simulink model "MDCC"  (R2021b)
settings: Solver=FixedStepDiscrete  StartTime=0.0  StopTime=10.0  FixedStep=0.0001  RelTol=1e-3
model workspace (MATLAB code in the model file):
  | cmdLim = Simulink.Parameter;
  | cmdLim.Value = 15;
  | cmdLim.Description = 'Limit for controlling the maximum surface command angle.';
  | cmdLim.Min = 0;
  | cmdLim.Max = 90;
  | cmdLim.DocUnits = 'deg';
  | 
  | dispGain = Simulink.Parameter;
  | dispGain.Value = 0.75;
  | dispGain.Description = 'Gain applied to the displacement error.';
  | dispGain.Min = 0;
  | dispGain.Max = [];
  | dispGain.DocUnits = 'deg/sec/deg';
  | 
  | dispLim = Simulink.Parameter;
  | dispLim.Value = 30;
  | dispLim.Description = 'Limit for controlling the maximum commanded angle.';
  | dispLim.Min = 0;
  | dispLim.Max = 180;
  | dispLim.DocUnits = 'deg';
  | 
  | intGain = Simulink.Parameter;
  | intGain.Value = 0.5;
  | intGain.Description = 'Gain applied to the integral error.';
  | intGain.Min = 0;
  | intGain.Max = [];
  | intGain.DocUnits = 'deg/sec/deg/sec';
  | 
  | intLim = Simulink.Parameter;
  | intLim.Value = 5;
  | intLim.Description = 'Limit for controlling the maximum commanded angle.';
  | intLim.Min = 0;
  | intLim.Max = 90;
  | intLim.DocUnits = 'deg';
  | 
  | rateGain = Simulink.Parameter;
  | rateGain.Value = 2;
  | rateGain.Description = 'Gain applied to the rate error.';
  | rateGain.Min = 0;
  | rateGain.Max = [];
  | rateGain.DocUnits = 'deg/deg/sec';
  | 
  | rateLim = Simulink.Parameter;
  | rateLim.Value = 6;
  | rateLim.Description = 'Limit for controlling the maximum commanded angle.';
  | rateLim.Min = 0;
  | rateLim.Max = 180;
  | rateLim.DocUnits = 'deg/sec';
  | 
  | hdgGain = Simulink.Parameter;
  | hdgGain.Value = 0.015;
values from neighbouring files (symbols this model uses):
  KfDeadCompen_SetDeltaTime_us = myPackage.Parameter    [DeadCompen.m]
  Ts = 5E-6    (= 5e-06)    [iPMSM_data.m]
  VbDeadComp_SwtUseIsttrDes_flg = myPackage.Parameter    [DeadCompen.m]
  VfDeadCompen_ISttrDdeThdSwt_A = myPackage.Parameter    [DeadCompen.m]
  VfDeadCompen_ISttrIgbtThdSwt_A = myPackage.Parameter    [DeadCompen.m]
  VfDeadCompen_rDdeISttrHi_R = myPackage.Parameter    [DeadCompen.m]
  VfDeadCompen_rDdeISttrLo_R = myPackage.Parameter    [DeadCompen.m]
  VfDeadCompen_rIgbtISttrHi_R = myPackage.Parameter    [DeadCompen.m]
  VfDeadCompen_rIgbtISttrLo_R = myPackage.Parameter    [DeadCompen.m]
  VfDeadCompen_uDdeISttrHi_V = myPackage.Parameter    [DeadCompen.m]
  VfDeadCompen_uDdeISttrLo_V = myPackage.Parameter    [DeadCompen.m]
  VfDeadCompen_uIgbtISttrHi_V = myPackage.Parameter    [DeadCompen.m]
  VfDeadCompen_uIgbtISttrLo_V = myPackage.Parameter    [DeadCompen.m]
undefined symbols (not defined in the file or in its folder): CosTable12bit_Y, GLBCal_GLBCal_Kf_DCLinkOverVolErrThd_V, GLBCal_GLBCal_Kf_DCLinkUnderVolErrThd_V, GLBCal_GLBCal_Kf_EquiLd_NULL, GLBCal_GLBCal_Kf_EquiLq_NULL, GLBCal_GLBCal_Kf_MotorRatedSpeed_rpm, GLBCal_GLBCal_Kf_MotorSpeedHysteresis_Coef, GLBCal_Ke_MotorPolePairsNum_NULL, IoHwAbOpArg_PwmDutyCyclePhU_NULL, IoHwAbOpArg_PwmDutyCyclePhV_NULL, IoHwAbOpArg_PwmDutyCyclePhW_NULL, IoHwAbOpArg_PwmOutputEn, KbMDCC_DeadTimeCompEn_flg, KbMDCC_MCF_flgHarmInIsdqTab11ZR_flg, KbMDCC_MCF_flgHarmInIsdqTab13ZR_flg, KbMDCC_MCF_flgHarmInIsdqTab5ZR_flg, KbMDCC_MCF_flgHarmInIsdqTab7ZR_flg, KbMDCC_MCF_flgHarmInject_flg, KbMDCC_SetEAngleEn_flg, KbMDCC_UdUqFwOmit_flg, KfDeadCompen_CpPeriodTimesT_NULL, KfMDCC_ActiveDischargeIdCurVal_A, KfMDCC_ActiveDischargeIqCurVal_A, KfMDCC_DCLinkVolRate_coef, KfMDCC_DebugEAngleInit_rad, KfMDCC_DebugUalphaVolCmd_V, KfMDCC_DebugUbetaVolCmd_V, KfMDCC_DebugUdCmd_V, KfMDCC_DebugUqCmd_V, KfMDCC_DebugUsCmd_V, KfMDCC_DebugUsRate_V, KfMDCC_IMCResp_NULL, KfMDCC_IMCStab_NULL, KfMDCC_InvParkCpPeriodTimesT_NULL, KfMDCC_MCF_CircAge_NULL, KfMDCC_MCF_flgUse11Harm_flg, KfMDCC_MCF_flgUse13Harm_flg, KfMDCC_MCF_flgUse5Harm_flg, KfMDCC_MCF_flgUse7Harm_flg, KfMDCC_MCF_Harm1113FLParamSpeedThrd_rads, KfMDCC_MCF_Harm57FLParamSpeedThrd_rads, KfMDCC_MCF_HarmcofFltN_NULL, KfMDCC_MCF_HarmCpnAg_NULL, KfMDCC_MCF_HarmfLParaHigh_coef, KfMDCC_MCF_HarmfLParaLow_coef, KfMDCC_MCF_HarmIn1113ZRY_Trq_Nm, KfMDCC_MCF_HarmIn11_SpdLimHigh_rads, KfMDCC_MCF_HarmIn11_SpdLimLow_rads, KfMDCC_MCF_HarmIn11ZRY_Isd_A, KfMDCC_MCF_HarmIn11ZRY_Isq_A, KfMDCC_MCF_HarmIn13_SpdLimHigh_rads, KfMDCC_MCF_HarmIn13_SpdLimLow_rads, KfMDCC_MCF_HarmIn13ZRY_Isd_A, KfMDCC_MCF_HarmIn13ZRY_Isq_A, KfMDCC_MCF_HarmIn57ZRY_Trq_Nm, KfMDCC_MCF_HarmIn5_SpdLimHigh_rads, KfMDCC_MCF_HarmIn5_SpdLimLow_rads, KfMDCC_MCF_HarmIn5ZRY_Isd_A, KfMDCC_MCF_HarmIn5ZRY_Isq_A, KfMDCC_MCF_HarmIn7_SpdLimHigh_rads ... (+47)
libraries: simulink x40, PMSM_Library x3, mcbcontrolslib x1
(part 6 of 8)

== system MDCC/DoCurCtr_sys/MDCC/SVM_Calc/DeadComp_Sys/DeadCur_Calc/N_Select_Calc/Subsystem2/Subsystem ==
  VfPwmFreq_Hz : Inport
  Add5 : Sum  Commented=on
  Divide : Product  Inputs=*/
  KfDeadCompen_CpPeriodTimesT_NULL : Constant  Value=KfDeadCompen_CpPeriodTimesT_NULL  OutDataTypeStr=single
  KfMDCC_InvParkCpPeriodTimesT_NULL : Constant  Commented=on  Value=KfMDCC_InvParkCpPeriodTimesT_NULL
  TimeComp : Outport
  wires:
  VfPwmFreq_Hz/1 -> Divide/2
  Divide/1 -> TimeComp/1
  KfDeadCompen_CpPeriodTimesT_NULL/1 -> Divide/1

== system MDCC/DoCurCtr_sys/MDCC/SVM_Calc/DeadComp_Sys/DeadTime_Calc/Tavon_Calc/ia/If Action Subsystem ==
  Phase_Dyc : Inport
  uIgbt : Inport  Port=2
  uDde : Inport  Port=3
  uDcLink : Inport  Port=4
  Action Port : ActionPort  ActionPortLabel=if(u1 == 1)
  Add : Sum  Inputs=-+
  Add1 : Sum  Inputs=+-
  Add2 : Sum  Inputs=--+
  Constant : Constant  OutDataTypeStr=single
  Divide : Product  Inputs=*/
  Product : Product
  Product1 : Product
  "dycCorr " : Outport
  wires:
  Phase_Dyc/1 -> Product/1, Add/1
  uIgbt/1 -> Product/2, Add2/1
  uDde/1 -> Add2/2, Product1/2
  Add/1 -> Product1/1
  Constant/1 -> Add/2
  Product/1 -> Add1/1
  Product1/1 -> Add1/2
  uDcLink/1 -> Add2/3
  Add1/1 -> Divide/1
  Add2/1 -> Divide/2
  Divide/1 -> "dycCorr "/1

== system MDCC/DoCurCtr_sys/MDCC/SVM_Calc/DeadComp_Sys/DeadTime_Calc/Tavon_Calc/ia/If Action Subsystem1 ==
  Phase_Dyc : Inport
  uIgbt : Inport  Port=2
  uDde : Inport  Port=3
  uDcLink : Inport  Port=4
  Action Port : ActionPort  ActionPortLabel=else
  Add : Sum  Inputs=-+
  Add1 : Sum  Inputs=+-
  Add2 : Sum  Inputs=--+
  Constant : Constant  OutDataTypeStr=single
  Divide : Product  Inputs=*/
  Product : Product
  Product1 : Product
  "dycCorr " : Outport
  wires:
  Phase_Dyc/1 -> Product/1, Add/1
  uDde/1 -> Add2/1, Product/2
  uIgbt/1 -> Add2/2, Product1/2
  Add/1 -> Product1/1
  Constant/1 -> Add/2
  Product/1 -> Add1/1
  Product1/1 -> Add1/2
  uDcLink/1 -> Add2/3
  Add1/1 -> Divide/1
  Add2/1 -> Divide/2
  Divide/1 -> "dycCorr "/1

== system MDCC/DoCurCtr_sys/MDCC/SVM_Calc/DeadComp_Sys/DeadTime_Calc/Tavon_Calc/ia/uDdeCalc ==
  iPhaseAbs : Inport
  Compare To Constant : simulink/Logic and Bit Operations/Compare To Constant  relop=<  const=VfDeadCompen_ISttrDdeThdSwt_A  OutDataTypeStr=boolean
  If : If  IfExpression=u1 == 1
  If Action Subsystem : Subsystem  TreatAsAtomicUnit=on
  If Action Subsystem1 : Subsystem  TreatAsAtomicUnit=on
  Merge : Merge
  uDde : Outport
  wires:
  iPhaseAbs/1 -> [A], Compare To Constant/1
  If/2 -> If Action Subsystem1/Action
  Merge/1 -> uDde/1
  If/1 -> If Action Subsystem/Action
  If Action Subsystem/1(UDde) -> Merge/1
  Compare To Constant/1 -> If/1
  If Action Subsystem1/1(UDde) -> Merge/2
  [A] -> If Action Subsystem/1(iPhaseAbs)
  [A] -> If Action Subsystem1/1(iPhaseAbs)

== system MDCC/DoCurCtr_sys/MDCC/SVM_Calc/DeadComp_Sys/DeadTime_Calc/Tavon_Calc/ia/uIgbtCalc ==
  iPhaseAbs : Inport
  Compare To Constant : simulink/Logic and Bit Operations/Compare To Constant  relop=<  const=VfDeadCompen_ISttrIgbtThdSwt_A  OutDataTypeStr=boolean
  If : If  IfExpression=u1 == 0
  If Action Subsystem : Subsystem  TreatAsAtomicUnit=on
  If Action Subsystem1 : Subsystem  TreatAsAtomicUnit=on
  Merge : Merge
  uIgbt : Outport
  wires:
  iPhaseAbs/1 -> Compare To Constant/1, [B]
  If/2 -> If Action Subsystem1/Action
  Merge/1 -> uIgbt/1
  If/1 -> If Action Subsystem/Action
  If Action Subsystem/1(uIgbt) -> Merge/1
  Compare To Constant/1 -> If/1
  If Action Subsystem1/1(uIgbt) -> Merge/2
  [B] -> If Action Subsystem/1(iPhaseAbs)
  [B] -> If Action Subsystem1/1(iPhaseAbs)

== system MDCC/DoCurCtr_sys/MDCC/SVM_Calc/DeadComp_Sys/DeadTime_Calc/Tavon_Calc/ib/If Action Subsystem ==
  Phase_Dyc : Inport
  uIgbt : Inport  Port=2
  uDde : Inport  Port=3
  uDcLink : Inport  Port=4
  Action Port : ActionPort  ActionPortLabel=if(u1 == 1)
  Add : Sum  Inputs=-+
  Add1 : Sum  Inputs=+-
  Add2 : Sum  Inputs=--+
  Constant : Constant  OutDataTypeStr=single
  Divide : Product  Inputs=*/
  Product : Product
  Product1 : Product
  "dycCorr " : Outport
  wires:
  Phase_Dyc/1 -> Product/1, Add/1
  uIgbt/1 -> Product/2, Add2/1
  uDde/1 -> Add2/2, Product1/2
  Add/1 -> Product1/1
  Constant/1 -> Add/2
  Product/1 -> Add1/1
  Product1/1 -> Add1/2
  uDcLink/1 -> Add2/3
  Add1/1 -> Divide/1
  Add2/1 -> Divide/2
  Divide/1 -> "dycCorr "/1

== system MDCC/DoCurCtr_sys/MDCC/SVM_Calc/DeadComp_Sys/DeadTime_Calc/Tavon_Calc/ib/If Action Subsystem1 ==
  Phase_Dyc : Inport
  uIgbt : Inport  Port=2
  uDde : Inport  Port=3
  uDcLink : Inport  Port=4
  Action Port : ActionPort  ActionPortLabel=else
  Add : Sum  Inputs=-+
  Add1 : Sum  Inputs=+-
  Add2 : Sum  Inputs=--+
  Constant : Constant  OutDataTypeStr=single
  Divide : Product  Inputs=*/
  Product : Product
  Product1 : Product
  "dycCorr " : Outport
  wires:
  Phase_Dyc/1 -> Product/1, Add/1
  uDde/1 -> Add2/1, Product/2
  uIgbt/1 -> Add2/2, Product1/2
  Add/1 -> Product1/1
  Constant/1 -> Add/2
  Product/1 -> Add1/1
  Product1/1 -> Add1/2
  uDcLink/1 -> Add2/3
  Add1/1 -> Divide/1
  Add2/1 -> Divide/2
  Divide/1 -> "dycCorr "/1

== system MDCC/DoCurCtr_sys/MDCC/SVM_Calc/DeadComp_Sys/DeadTime_Calc/Tavon_Calc/ib/uDdeCalc ==
  iPhaseAbs : Inport
  Compare To Constant : simulink/Logic and Bit Operations/Compare To Constant  relop=<  const=VfDeadCompen_ISttrDdeThdSwt_A  OutDataTypeStr=boolean
  If : If  IfExpression=u1 == 1
  If Action Subsystem : Subsystem  TreatAsAtomicUnit=on
  If Action Subsystem1 : Subsystem  TreatAsAtomicUnit=on
  Merge : Merge
  uDde : Outport
  wires:
  iPhaseAbs/1 -> [A], Compare To Constant/1
  If/2 -> If Action Subsystem1/Action
  Merge/1 -> uDde/1
  If/1 -> If Action Subsystem/Action
  If Action Subsystem/1(UDde) -> Merge/1
  Compare To Constant/1 -> If/1
  If Action Subsystem1/1(UDde) -> Merge/2
  [A] -> If Action Subsystem/1(iPhaseAbs)
  [A] -> If Action Subsystem1/1(iPhaseAbs)

== system MDCC/DoCurCtr_sys/MDCC/SVM_Calc/DeadComp_Sys/DeadTime_Calc/Tavon_Calc/ib/uIgbtCalc ==
  iPhaseAbs : Inport
  Compare To Constant : simulink/Logic and Bit Operations/Compare To Constant  relop=<  const=VfDeadCompen_ISttrIgbtThdSwt_A  OutDataTypeStr=boolean
  If : If  IfExpression=u1 == 0
  If Action Subsystem : Subsystem  TreatAsAtomicUnit=on
  If Action Subsystem1 : Subsystem  TreatAsAtomicUnit=on
  Merge : Merge
  uIgbt : Outport
  wires:
  iPhaseAbs/1 -> Compare To Constant/1, [B]
  If/2 -> If Action Subsystem1/Action
  Merge/1 -> uIgbt/1
  If/1 -> If Action Subsystem/Action
  If Action Subsystem/1(uIgbt) -> Merge/1
  Compare To Constant/1 -> If/1
  If Action Subsystem1/1(uIgbt) -> Merge/2
  [B] -> If Action Subsystem/1(iPhaseAbs)
  [B] -> If Action Subsystem1/1(iPhaseAbs)

== system MDCC/DoCurCtr_sys/MDCC/SVM_Calc/DeadComp_Sys/DeadTime_Calc/Tavon_Calc/ic/If Action Subsystem ==
  Phase_Dyc : Inport
  uIgbt : Inport  Port=2
  uDde : Inport  Port=3
  uDcLink : Inport  Port=4
  Action Port : ActionPort  ActionPortLabel=if(u1 == 1)
  Add : Sum  Inputs=-+
  Add1 : Sum  Inputs=+-
  Add2 : Sum  Inputs=--+
  Constant : Constant  OutDataTypeStr=single
  Divide : Product  Inputs=*/
  Product : Product
  Product1 : Product
  "dycCorr " : Outport
  wires:
  Phase_Dyc/1 -> Product/1, Add/1
  uIgbt/1 -> Product/2, Add2/1
  uDde/1 -> Add2/2, Product1/2
  Add/1 -> Product1/1
  Constant/1 -> Add/2
  Product/1 -> Add1/1
  Product1/1 -> Add1/2
  uDcLink/1 -> Add2/3
  Add1/1 -> Divide/1
  Add2/1 -> Divide/2
  Divide/1 -> "dycCorr "/1

== system MDCC/DoCurCtr_sys/MDCC/SVM_Calc/DeadComp_Sys/DeadTime_Calc/Tavon_Calc/ic/If Action Subsystem1 ==
  Phase_Dyc : Inport
  uIgbt : Inport  Port=2
  uDde : Inport  Port=3
  uDcLink : Inport  Port=4
  Action Port : ActionPort  ActionPortLabel=else
  Add : Sum  Inputs=-+
  Add1 : Sum  Inputs=+-
  Add2 : Sum  Inputs=--+
  Constant : Constant  OutDataTypeStr=single
  Divide : Product  Inputs=*/
  Product : Product
  Product1 : Product
  "dycCorr " : Outport
  wires:
  Phase_Dyc/1 -> Product/1, Add/1
  uDde/1 -> Add2/1, Product/2
  uIgbt/1 -> Add2/2, Product1/2
  Add/1 -> Product1/1
  Constant/1 -> Add/2
  Product/1 -> Add1/1
  Product1/1 -> Add1/2
  uDcLink/1 -> Add2/3
  Add1/1 -> Divide/1
  Add2/1 -> Divide/2
  Divide/1 -> "dycCorr "/1

== system MDCC/DoCurCtr_sys/MDCC/SVM_Calc/DeadComp_Sys/DeadTime_Calc/Tavon_Calc/ic/uDdeCalc ==
  iPhaseAbs : Inport
  Compare To Constant : simulink/Logic and Bit Operations/Compare To Constant  relop=<  const=VfDeadCompen_ISttrDdeThdSwt_A  OutDataTypeStr=boolean
  If : If  IfExpression=u1 == 1
  If Action Subsystem : Subsystem  TreatAsAtomicUnit=on
  If Action Subsystem1 : Subsystem  TreatAsAtomicUnit=on
  Merge : Merge
  uDde : Outport
  wires:
  iPhaseAbs/1 -> [A], Compare To Constant/1
  If/2 -> If Action Subsystem1/Action
  Merge/1 -> uDde/1
  If/1 -> If Action Subsystem/Action
  If Action Subsystem/1(UDde) -> Merge/1
  Compare To Constant/1 -> If/1
  If Action Subsystem1/1(UDde) -> Merge/2
  [A] -> If Action Subsystem/1(iPhaseAbs)
  [A] -> If Action Subsystem1/1(iPhaseAbs)

== system MDCC/DoCurCtr_sys/MDCC/SVM_Calc/DeadComp_Sys/DeadTime_Calc/Tavon_Calc/ic/uIgbtCalc ==
  iPhaseAbs : Inport
  Compare To Constant : simulink/Logic and Bit Operations/Compare To Constant  relop=<  const=VfDeadCompen_ISttrIgbtThdSwt_A  OutDataTypeStr=boolean
  If : If  IfExpression=u1 == 0
  If Action Subsystem : Subsystem  TreatAsAtomicUnit=on
  If Action Subsystem1 : Subsystem  TreatAsAtomicUnit=on
  Merge : Merge
  uIgbt : Outport
  wires:
  iPhaseAbs/1 -> Compare To Constant/1, [B]
  If/2 -> If Action Subsystem1/Action
  Merge/1 -> uIgbt/1
  If/1 -> If Action Subsystem/Action
  If Action Subsystem/1(uIgbt) -> Merge/1
  Compare To Constant/1 -> If/1
  If Action Subsystem1/1(uIgbt) -> Merge/2
  [B] -> If Action Subsystem/1(iPhaseAbs)
  [B] -> If Action Subsystem1/1(iPhaseAbs)

== system MDCC/DoCurCtr_sys/MDCC/SVM_Calc/MDSA/SVM_PU/T1_T2_Calc/Subsystem1/Enabled Subsystem ==
  Z : Inport
  Y : Inport  Port=2
  Action Port : ActionPort  ActionPortLabel=case [ 1 ]:
  T4 : Outport
  T6 : Outport  Port=2
  wires:
  Z/1 -> T4/1
  Y/1 -> T6/1

== system MDCC/DoCurCtr_sys/MDCC/SVM_Calc/MDSA/SVM_PU/T1_T2_Calc/Subsystem1/Enabled Subsystem1 ==
  Y : Inport
  X : Inport  Port=2
  Action Port : ActionPort  ActionPortLabel=case [ 2 ]:
  Gain : Gain  Gain=-1
  T4 : Outport
  T6 : Outport  Port=2
  wires:
  Y/1 -> T4/1
  Gain/1 -> T6/1
  X/1 -> Gain/1

== system MDCC/DoCurCtr_sys/MDCC/SVM_Calc/MDSA/SVM_PU/T1_T2_Calc/Subsystem1/Enabled Subsystem2 ==
  Z : Inport
  X : Inport  Port=2
  Action Port : ActionPort  ActionPortLabel=case [ 3 ]:
  Gain : Gain  Gain=-1
  T4 : Outport
  T6 : Outport  Port=2
  wires:
  Z/1 -> Gain/1
  X/1 -> T6/1
  Gain/1 -> T4/1

== system MDCC/DoCurCtr_sys/MDCC/SVM_Calc/MDSA/SVM_PU/T1_T2_Calc/Subsystem1/Enabled Subsystem3 ==
  X : Inport
  Z : Inport  Port=2
  Action Port : ActionPort  ActionPortLabel=case [ 4 ]:
  Gain : Gain  Gain=-1
  T4 : Outport
  T6 : Outport  Port=2
  wires:
  X/1 -> Gain/1
  Z/1 -> T6/1
  Gain/1 -> T4/1

== system MDCC/DoCurCtr_sys/MDCC/SVM_Calc/MDSA/SVM_PU/T1_T2_Calc/Subsystem1/Enabled Subsystem4 ==
  X : Inport
  Y : Inport  Port=2
  Action Port : ActionPort  ActionPortLabel=case [ 5 ]:
  Gain : Gain  Gain=-1
  T4 : Outport
  T6 : Outport  Port=2
  wires:
  Y/1 -> Gain/1
  X/1 -> T4/1
  Gain/1 -> T6/1

== system MDCC/DoCurCtr_sys/MDCC/SVM_Calc/MDSA/SVM_PU/T1_T2_Calc/Subsystem1/Enabled Subsystem5 ==
  Y : Inport
  Z : Inport  Port=2
  Action Port : ActionPort  ActionPortLabel=case [ 6 ]:
  Gain : Gain  Gain=-1
  Gain1 : Gain  Gain=-1
  T4 : Outport
  T6 : Outport  Port=2
  wires:
  Y/1 -> Gain/1
  Z/1 -> Gain1/1
  Gain/1 -> T4/1
  Gain1/1 -> T6/1

== system MDCC/DoCurCtr_sys/MDCC/SVM_Calc/MDSA/SVM_PU/T1_T2_Calc/Subsystem1/Enabled Subsystem6 ==
  Y : Inport
  Z : Inport  Port=2
  Action Port : ActionPort  ActionPortLabel=default:
  Gain : Gain  Gain=-1
  Gain1 : Gain  Gain=-1
  T4 : Outport
  T6 : Outport  Port=2
  wires:
  Y/1 -> Gain/1
  Z/1 -> Gain1/1
  Gain/1 -> T4/1
  Gain1/1 -> T6/1

== system MDCC/DoCurCtr_sys/MDCC/SVM_Calc/MDSA/SVM_PU/T1_T2_Calc/Subsystem2/If Action Subsystem ==
  Bus_T4T6 : Inport
  Action Port : ActionPort  ActionPortLabel=else
  Bus Selector : BusSelector  OutputSignals=T4,T6
  Signal Copy1 : SignalConversion  OverrideOpt=off
  Signal Copy2 : SignalConversion  OverrideOpt=off
  T1 : Outport
  T2 : Outport  Port=2
  wires:
  Bus_T4T6/1 -> Bus Selector/1
  Bus Selector/1 -> Signal Copy1/1  "<T4>"
  Bus Selector/2 -> Signal Copy2/1  "<T6>"
  Signal Copy1/1 -> T1/1
  Signal Copy2/1 -> T2/1

== system MDCC/DoCurCtr_sys/MDCC/SVM_Calc/MDSA/SVM_PU/T1_T2_Calc/Subsystem2/If Action Subsystem1 ==
  Bus_T4T6 : Inport
  Action Port : ActionPort  ActionPortLabel=elseif(u1 > 1)
  Add : Sum
  Bus Selector : BusSelector  OutputSignals=T4,T6
  Divide : Product  Inputs=*/
  Divide1 : Product  Inputs=/*
  T1 : Outport
  T2 : Outport  Port=2
  wires:
  Bus_T4T6/1 -> Bus Selector/1
  Bus Selector/1 -> Divide/1, Add/1  "<T4>"
  Bus Selector/2 -> Divide1/2, Add/2  "<T6>"
  Add/1 -> Divide1/1, Divide/2
  Divide/1 -> T1/1  "T1"
  Divide1/1 -> T2/1  "T2"

== system MDCC/DoCurCtr_sys/MDCC/SVM_Calc/MDSA/SVM_PU/T1_T2_Calc/Subsystem2/If Action Subsystem2 ==
  Bus_T4T6 : Inport
  Action Port : ActionPort  ActionPortLabel=if(u1 > 1.154 )
  Add1 : Sum
  Add2 : Sum  Inputs=++-
  Bus Selector1 : BusSelector  OutputSignals=T4,T6
  Constant : Constant  Value=1.154  OutDataTypeStr=single
  Divide : Product  Inputs=*/
  Divide1 : Product  Inputs=/*
  If Action Subsystem2 : Subsystem  TreatAsAtomicUnit=on
  If Action Subsystem3 : Subsystem  TreatAsAtomicUnit=on
  If1 : If  IfExpression=u1 ~= 0
  Merge2 : Merge
  Merge3 : Merge
  Relational Operator1 : RelationalOperator  OutDataTypeStr=boolean  RndMeth=Simplest
  T1 : Outport
  T2 : Outport  Port=2
  wires:
  Bus_T4T6/1 -> Bus Selector1/1
  Bus Selector1/2 -> Divide1/2, Add2/2, Add1/2  "<T6>"
  Divide/1 -> [T4_m], Relational Operator1/1  "T4_m"
  Bus Selector1/1 -> Divide/1, Add2/1, Add1/1  "<T4>"
  Divide1/1 -> [T6_m], Relational Operator1/2  "T6_m"
  Add1/1 -> Divide1/1, Divide/2
  Relational Operator1/1 -> If1/1
  Constant/1 -> Add2/3
  Add2/1 -> If Action Subsystem2/3(delta), If Action Subsystem3/3(delta)  "delta"
  If1/1 -> If Action Subsystem2/Action
  If1/2 -> If Action Subsystem3/Action
  If Action Subsystem2/1(T1) -> Merge2/1
  If Action Subsystem3/1(T1) -> Merge2/2
  If Action Subsystem3/2(T2) -> Merge3/2
  If Action Subsystem2/2(T2) -> Merge3/1
  Merge2/1 -> T1/1  "T1"
  Merge3/1 -> T2/1  "T2"
  [T4_m] -> If Action Subsystem3/1(T4_m), If Action Subsystem2/1(T4_m)
  [T6_m] -> If Action Subsystem3/2(T6_m), If Action Subsystem2/2(T6_m)

== system MDCC/DoCurCtr_sys/MDCC/SVM_Calc/MDSA/SVPWM/vIntp_PWMFOC_CalSec/CalABC/CalA ==
  In1 : Inport
  Constant : Constant
  Constant1 : Constant  Value=0
  Data Type Conversion : DataTypeConversion
  Data Type Conversion1 : DataTypeConversion
  Switch : Switch  Criteria=u2 > Threshold  ZeroCross=off
  A : Outport
  wires:
  Switch/1 -> A/1
  Data Type Conversion1/1 -> Switch/3
  Data Type Conversion/1 -> Switch/1
  Constant1/1 -> Data Type Conversion1/1
  Constant/1 -> Data Type Conversion/1
  In1/1 -> Switch/2

== system MDCC/DoCurCtr_sys/MDCC/SVM_Calc/MDSA/SVPWM/vIntp_PWMFOC_CalSec/CalABC/CalB ==
  In1 : Inport
  Constant : Constant
  Constant1 : Constant  Value=0
  Data Type Conversion : DataTypeConversion
  Data Type Conversion1 : DataTypeConversion
  Switch : Switch  Criteria=u2 > Threshold  ZeroCross=off
  B : Outport
  wires:
  In1/1 -> Switch/2
  Constant/1 -> Data Type Conversion/1
  Constant1/1 -> Data Type Conversion1/1
  Data Type Conversion/1 -> Switch/1
  Data Type Conversion1/1 -> Switch/3
  Switch/1 -> B/1

== system MDCC/DoCurCtr_sys/MDCC/SVM_Calc/MDSA/SVPWM/vIntp_PWMFOC_CalSec/CalABC/CalC ==
  In1 : Inport
  Constant : Constant
  Constant1 : Constant  Value=0
  Data Type Conversion : DataTypeConversion
  Data Type Conversion1 : DataTypeConversion
  Switch : Switch  Criteria=u2 > Threshold  ZeroCross=off
  C : Outport
  wires:
  Switch/1 -> C/1
  Data Type Conversion1/1 -> Switch/3
  Data Type Conversion/1 -> Switch/1
  Constant1/1 -> Data Type Conversion1/1
  Constant/1 -> Data Type Conversion/1
  In1/1 -> Switch/2

== system MDCC/DoCurCtr_sys/MDCC/SVM_Calc/MDSA/SVPWM/vIntp_PWMFOC_CalSec/CalVaVbVc/CalVa ==
  In1 : Inport
  Bus Selector : BusSelector  OutputSignals=Ubeta
  Va : Outport
  wires:
  Bus Selector/1 -> Va/1  "<Ubeta>"
  In1/1 -> Bus Selector/1

== system MDCC/DoCurCtr_sys/MDCC/SVM_Calc/MDSA/SVPWM/vIntp_PWMFOC_CalSec/CalVaVbVc/CalVb ==
  In1 : Inport
  1/2 : Constant  Value=0.5
  Add : Sum  Inputs=+-
  Bus Selector : BusSelector  OutputSignals=Ualpha,Ubeta
  Data Type Conversion : DataTypeConversion
  Data Type Conversion1 : DataTypeConversion
  Data Type Conversion2 : DataTypeConversion
  Product1 : Product
  Product2 : Product
  Sqrt(3)/2 : Constant  Value=0.866025
  Vb : Outport
  wires:
  Data Type Conversion2/1 -> Vb/1
  Product1/1 -> Add/2
  Product2/1 -> Add/1
  Data Type Conversion1/1 -> Product1/2
  Bus Selector/1 -> Product2/1  "<Ualpha>"
  1/2/1 -> Data Type Conversion1/1
  Data Type Conversion/1 -> Product2/2
  Sqrt(3)/2/1 -> Data Type Conversion/1
  Add/1 -> Data Type Conversion2/1
  Bus Selector/2 -> Product1/1  "<Ubeta>"
  In1/1 -> Bus Selector/1

== system MDCC/DoCurCtr_sys/MDCC/SVM_Calc/MDSA/SVPWM/vIntp_PWMFOC_CalSec/CalVaVbVc/CalVc ==
  In1 : Inport
  -1/2 : Constant  Value=-0.5
  -Sqrt(3)/2 : Constant  Value=-0.866025
  Add : Sum
  Bus Selector : BusSelector  OutputSignals=Ualpha,Ubeta
  Data Type Conversion : DataTypeConversion
  Data Type Conversion1 : DataTypeConversion
  Data Type Conversion2 : DataTypeConversion
  Product1 : Product
  Product2 : Product
  Vc : Outport
  wires:
  Data Type Conversion2/1 -> Vc/1
  Product1/1 -> Add/2
  Product2/1 -> Add/1
  Data Type Conversion1/1 -> Product1/2
  Bus Selector/1 -> Product2/1  "<Ualpha>"
  -1/2/1 -> Data Type Conversion1/1
  Data Type Conversion/1 -> Product2/2
  -Sqrt(3)/2/1 -> Data Type Conversion/1
  Add/1 -> Data Type Conversion2/1
  Bus Selector/2 -> Product1/1  "<Ubeta>"
  In1/1 -> Bus Selector/1

== system MDCC/DoCurCtr_sys/MDCC/SVM_Calc/MDSA/SVPWM/vIntp_PWMFOC_CalTriCompValue/CalCMPValue/Sec1 ==
  Bus_Tabc_IN : Inport
  Action Port : ActionPort  ActionPortLabel=case [ 1 ]:
  Bus Creator1 : BusCreator  Inputs=3
  Bus Selector : BusSelector  OutputSignals=signal2,signal1,signal3
  Signal Conversion : SignalConversion  OverrideOpt=off
  Signal Conversion1 : SignalConversion  OverrideOpt=off
  Signal Conversion2 : SignalConversion  OverrideOpt=off
  Bus_CMP : Outport
  wires:
  Signal Conversion2/1 -> Bus Creator1/3
  Signal Conversion1/1 -> Bus Creator1/2
  Signal Conversion/1 -> Bus Creator1/1
  Bus Selector/3 -> Signal Conversion2/1  "<signal3>"
  Bus Selector/2 -> Signal Conversion1/1  "<signal1>"
  Bus Selector/1 -> Signal Conversion/1  "<signal2>"
  Bus Creator1/1 -> Bus_CMP/1
  Bus_Tabc_IN/1 -> Bus Selector/1

== system MDCC/DoCurCtr_sys/MDCC/SVM_Calc/MDSA/SVPWM/vIntp_PWMFOC_CalTriCompValue/CalCMPValue/Sec2 ==
  Bus_Tabc_IN : Inport
  Action Port : ActionPort  ActionPortLabel=case [ 2 ]:
  Bus Creator : BusCreator  Inputs=3
  Bus Selector : BusSelector  OutputSignals=signal1,signal3,signal2
  Signal Conversion : SignalConversion  OverrideOpt=off
  Signal Conversion1 : SignalConversion  OverrideOpt=off
  Signal Conversion2 : SignalConversion  OverrideOpt=off
  Bus_CMP : Outport
  wires:
  Signal Conversion2/1 -> Bus Creator/3
  Signal Conversion1/1 -> Bus Creator/2
  Signal Conversion/1 -> Bus Creator/1
  Bus_Tabc_IN/1 -> Bus Selector/1
  Bus Selector/3 -> Signal Conversion2/1  "<signal2>"
  Bus Selector/2 -> Signal Conversion1/1  "<signal3>"
  Bus Selector/1 -> Signal Conversion/1  "<signal1>"
  Bus Creator/1 -> Bus_CMP/1

== system MDCC/DoCurCtr_sys/MDCC/SVM_Calc/MDSA/SVPWM/vIntp_PWMFOC_CalTriCompValue/CalCMPValue/Sec3 ==
  Bus_Tabc_IN : Inport
  Action Port : ActionPort  ActionPortLabel=case [ 3 ]:
  Bus Creator : BusCreator  Inputs=3
  Bus Selector : BusSelector  OutputSignals=signal1,signal2,signal3
  Signal Conversion : SignalConversion  OverrideOpt=off
  Signal Conversion1 : SignalConversion  OverrideOpt=off
  Signal Conversion2 : SignalConversion  OverrideOpt=off
  Bus_CMP : Outport
  wires:
  Signal Conversion2/1 -> Bus Creator/3
  Signal Conversion1/1 -> Bus Creator/2
  Signal Conversion/1 -> Bus Creator/1
  Bus Selector/3 -> Signal Conversion2/1  "<signal3>"
  Bus Selector/2 -> Signal Conversion1/1  "<signal2>"
  Bus Selector/1 -> Signal Conversion/1  "<signal1>"
  Bus_Tabc_IN/1 -> Bus Selector/1
  Bus Creator/1 -> Bus_CMP/1

== system MDCC/DoCurCtr_sys/MDCC/SVM_Calc/MDSA/SVPWM/vIntp_PWMFOC_CalTriCompValue/CalCMPValue/Sec4 ==
  Bus_Tabc_IN : Inport
  Action Port : ActionPort  ActionPortLabel=case [ 4 ]:
  Bus Creator : BusCreator  Inputs=3
  Bus Selector : BusSelector  OutputSignals=signal3,signal2,signal1
  Signal Conversion : SignalConversion  OverrideOpt=off
  Signal Conversion1 : SignalConversion  OverrideOpt=off
  Signal Conversion2 : SignalConversion  OverrideOpt=off
  Bus_CMP : Outport
  wires:
  Signal Conversion2/1 -> Bus Creator/3
  Signal Conversion1/1 -> Bus Creator/2
  Signal Conversion/1 -> Bus Creator/1
  Bus_Tabc_IN/1 -> Bus Selector/1
  Bus Selector/3 -> Signal Conversion2/1  "<signal1>"
  Bus Selector/2 -> Signal Conversion1/1  "<signal2>"
  Bus Selector/1 -> Signal Conversion/1  "<signal3>"
  Bus Creator/1 -> Bus_CMP/1

== system MDCC/DoCurCtr_sys/MDCC/SVM_Calc/MDSA/SVPWM/vIntp_PWMFOC_CalTriCompValue/CalCMPValue/Sec5 ==
  Bus_Tabc_IN : Inport
  Action Port : ActionPort  ActionPortLabel=case [ 5 ]:
  Bus Creator : BusCreator  Inputs=3
  Bus Selector : BusSelector  OutputSignals=signal3,signal1,signal2
  Signal Conversion : SignalConversion  OverrideOpt=off
  Signal Conversion1 : SignalConversion  OverrideOpt=off
  Signal Conversion2 : SignalConversion  OverrideOpt=off
  Bus_CMP : Outport
  wires:
  Signal Conversion2/1 -> Bus Creator/3
  Signal Conversion1/1 -> Bus Creator/2
  Signal Conversion/1 -> Bus Creator/1
  Bus_Tabc_IN/1 -> Bus Selector/1
  Bus Selector/3 -> Signal Conversion2/1  "<signal2>"
  Bus Selector/2 -> Signal Conversion1/1  "<signal1>"
  Bus Selector/1 -> Signal Conversion/1  "<signal3>"
  Bus Creator/1 -> Bus_CMP/1

== system MDCC/DoCurCtr_sys/MDCC/SVM_Calc/MDSA/SVPWM/vIntp_PWMFOC_CalTriCompValue/CalCMPValue/Sec6 ==
  Bus_Tabc_IN : Inport
  Action Port : ActionPort  ActionPortLabel=case [ 6 ]:
  Bus Creator : BusCreator  Inputs=3
  Bus Selector : BusSelector  OutputSignals=signal2,signal3,signal1
  Signal Conversion : SignalConversion  OverrideOpt=off
  Signal Conversion1 : SignalConversion  OverrideOpt=off
  Signal Conversion2 : SignalConversion  OverrideOpt=off
  Bus_CMP : Outport
  wires:
  Signal Conversion2/1 -> Bus Creator/3
  Signal Conversion1/1 -> Bus Creator/2
  Signal Conversion/1 -> Bus Creator/1
  Bus Selector/1 -> Signal Conversion/1  "<signal2>"
  Bus Selector/3 -> Signal Conversion2/1  "<signal1>"
  Bus Selector/2 -> Signal Conversion1/1  "<signal3>"
  Bus_Tabc_IN/1 -> Bus Selector/1
  Bus Creator/1 -> Bus_CMP/1

== system MDCC/DoCurCtr_sys/MDCC/SVM_Calc/MDSA/SVPWM/vIntp_PWMFOC_CalTriCompValue/CalTabc/Cal_T1T2 ==
  Bus_XYZ_IN : Inport
  N_VALUE_IN : Inport  Port=2
  Data Type Conversion : DataTypeConversion
  Merge : Merge  Inputs=6
  Sec1 : Subsystem
  Sec2 : Subsystem
  Sec3 : Subsystem
  Sec4 : Subsystem
  Sec5 : Subsystem
  Sec6 : Subsystem
  Switch Case : SwitchCase  CaseConditions={1,2,3,4,5,6}  ShowDefaultCase=off
  Bus_T1T2_OUT : Outport
  wires:
  Sec1/1(Bus_T1T2) -> Merge/1
  Sec6/1(Bus_T1T2) -> Merge/6
  Sec5/1(Bus_T1T2) -> Merge/5
  Sec2/1(Bus_T1T2) -> Merge/2
  Sec3/1(Bus_T1T2) -> Merge/3
  Sec4/1(Bus_T1T2) -> Merge/4
  [Cal_T1T2_Sec2] -> Sec2/Action
  [Cal_T1T2_Sec6] -> Sec6/Action
  [Cal_T1T2_Sec5] -> Sec5/Action
  [Cal_T1T2_Sec4] -> Sec4/Action
  [Cal_T1T2_Sec3] -> Sec3/Action
  [Cal_T1T2_Sec1] -> Sec1/Action
  Switch Case/6 -> [Cal_T1T2_Sec6]
  Switch Case/5 -> [Cal_T1T2_Sec5]
  Switch Case/4 -> [Cal_T1T2_Sec4]
  Switch Case/3 -> [Cal_T1T2_Sec3]
  Switch Case/2 -> [Cal_T1T2_Sec2]
  Switch Case/1 -> [Cal_T1T2_Sec1]
  Data Type Conversion/1 -> Switch Case/1
  Bus_XYZ_IN/1 -> Sec1/1(Bus_XYZ_IN), Sec2/1(Bus_XYZ_IN), Sec3/1(Bus_XYZ_IN), Sec4/1(Bus_XYZ_IN), Sec6/1(Bus_XYZ_IN), Sec5/1(Bus_XYZ_IN)
  N_VALUE_IN/1 -> Data Type Conversion/1
  Merge/1 -> Bus_T1T2_OUT/1

== system MDCC/DoCurCtr_sys/MDCC/SVM_Calc/MDSA/SVPWM/vIntp_PWMFOC_CalTriCompValue/CalTabc/Cal_TabcValue ==
  Bus_T1T2_IN : Inport
  Bus_Ts_Vdc : Inport  Port=2
  CalTabcValue : Subsystem
  ManageT1T2 : Subsystem
  Bus_Tabc : Outport
  wires:
  CalTabcValue/1(Bus_Tabc) -> Bus_Tabc/1
  ManageT1T2/1(Bus_T1T2_Adjusted) -> CalTabcValue/1(Bus_T1T2_Adjusted_IN)
  Bus_T1T2_IN/1 -> ManageT1T2/1(Bus_T1T2_IN)
  Bus_Ts_Vdc/1 -> ManageT1T2/2(Bus_Ts_Vdc), CalTabcValue/2(Bus_Ts_Vdc)

== system MDCC/DoCurCtr_sys/MDCC/SVM_Calc/MDSA/SVPWM/vIntp_PWMFOC_CalTriCompValue/CalXYZ/Cal_X ==
  Bus_UalphaUbeta : Inport
  Bus_Ts_Vdc : Inport  Port=2
  Bus Selector : BusSelector  OutputSignals=Ubeta
  Bus Selector1 : BusSelector  OutputSignals=Ts,Vdc
  Data Type Conversion{,1..4} (5 alike) : DataTypeConversion
  Divide : Product  Inputs=*/
  Product : Product
  Product1 : Product
  Sqrt(3) : Constant  Value=1.7320508
  X_Value : Outport
  wires:
  Data Type Conversion4/1 -> X_Value/1
  Data Type Conversion3/1 -> Product/1
  Data Type Conversion2/1 -> Divide/1
  Data Type Conversion1/1 -> Divide/2
  Data Type Conversion/1 -> Product/2
  Product1/1 -> Data Type Conversion4/1
  Bus Selector/1 -> Product1/1  "<Ubeta>"
  Product/1 -> Product1/2
  Divide/1 -> Data Type Conversion3/1
  Sqrt(3)/1 -> Data Type Conversion/1
  Bus_UalphaUbeta/1 -> Bus Selector/1
  Bus_Ts_Vdc/1 -> Bus Selector1/1
  Bus Selector1/1 -> Data Type Conversion2/1  "<Ts>"
  Bus Selector1/2 -> Data Type Conversion1/1  "<Vdc>"

== system MDCC/DoCurCtr_sys/MDCC/SVM_Calc/MDSA/SVPWM/vIntp_PWMFOC_CalTriCompValue/CalXYZ/Cal_Y ==
  Bus_UalphaUbeta : Inport
  Bus_Ts_Vdc : Inport  Port=2
  3/2 : Constant  Value=1.5
  Add : Sum
  Bus Selector : BusSelector  OutputSignals=Ualpha,Ubeta
  Bus Selector1 : BusSelector  OutputSignals=Ts,Vdc
  Constant2 : Constant
  Data Type Conversion{,1..6} (7 alike) : DataTypeConversion
  Divide : Product  Inputs=*/
  Divide1 : Product  Inputs=*/  OutDataTypeStr=single
  Product : Product
  Product1 : Product
  Product2 : Product
  Sqrt(3)/2 : Constant  Value=0.866025
  Y_Value : Outport
  wires:
  Data Type Conversion4/1 -> Divide1/2
  Product2/1 -> Y_Value/1
  Constant2/1 -> Data Type Conversion4/1
  Divide/1 -> Divide1/1
  Divide1/1 -> Data Type Conversion6/1
  Data Type Conversion3/1 -> Divide/1
  Data Type Conversion2/1 -> Divide/2
  Add/1 -> Data Type Conversion5/1
  Product/1 -> Add/2
  Product1/1 -> Add/1
  Bus Selector/1 -> Product1/1  "<Ualpha>"
  Data Type Conversion1/1 -> Product1/2
  3/2/1 -> Data Type Conversion1/1
  Bus Selector/2 -> Product/1  "<Ubeta>"
  Data Type Conversion/1 -> Product/2
  Sqrt(3)/2/1 -> Data Type Conversion/1
  Bus_UalphaUbeta/1 -> Bus Selector/1
  Data Type Conversion5/1 -> Product2/1
  Data Type Conversion6/1 -> Product2/2
  Bus_Ts_Vdc/1 -> Bus Selector1/1
  Bus Selector1/1 -> Data Type Conversion3/1  "<Ts>"
  Bus Selector1/2 -> Data Type Conversion2/1  "<Vdc>"

== system MDCC/DoCurCtr_sys/MDCC/SVM_Calc/MDSA/SVPWM/vIntp_PWMFOC_CalTriCompValue/CalXYZ/Cal_Z ==
  Bus_UalphaUbeta : Inport
  Bus_Ts_Vdc : Inport  Port=2
  3/2 : Constant  Value=1.5
  Add : Sum  Inputs=-+
  Bus Selector : BusSelector  OutputSignals=Ualpha,Ubeta
  Bus Selector1 : BusSelector  OutputSignals=Ts,Vdc
  Constant2 : Constant
  Data Type Conversion{,1..6} (7 alike) : DataTypeConversion
  Divide : Product  Inputs=*/
  Divide1 : Product  Inputs=*/
  Product : Product
  Product1 : Product
  Product2 : Product
  Sqrt(3)/2 : Constant  Value=0.866025
  Z_Value : Outport
  wires:
  Bus_UalphaUbeta/1 -> Bus Selector/1
  Sqrt(3)/2/1 -> Data Type Conversion/1
  Data Type Conversion/1 -> Product/2
  Bus Selector/2 -> Product/1  "<Ubeta>"
  3/2/1 -> Data Type Conversion1/1
  Data Type Conversion1/1 -> Product1/2
  Bus Selector/1 -> Product1/1  "<Ualpha>"
  Product1/1 -> Add/1
  Product/1 -> Add/2
  Add/1 -> Data Type Conversion5/1
  Data Type Conversion2/1 -> Divide/2
  Data Type Conversion3/1 -> Divide/1
  Divide1/1 -> Data Type Conversion6/1
  Divide/1 -> Divide1/1
  Constant2/1 -> Data Type Conversion4/1
  Product2/1 -> Z_Value/1
  Data Type Conversion4/1 -> Divide1/2
  Data Type Conversion5/1 -> Product2/1
  Data Type Conversion6/1 -> Product2/2
  Bus_Ts_Vdc/1 -> Bus Selector1/1
  Bus Selector1/1 -> Data Type Conversion3/1  "<Ts>"
  Bus Selector1/2 -> Data Type Conversion2/1  "<Vdc>"

== system MDCC/DoCurCtr_sys/MDCC/UdUqCalc_Sys/MDCC_MCF_Sys/Enabled Subsystem/Harmonic_Injection_11/Set_11_steps_current_isdqdes/LookUpEAngleCosSin1 ==
  VuMDCC_MotorPositionCnt_NULL : Inport  OutMin=[0]  OutMax=[4095]
  Constant2 : Constant  Value=CosTable12bit_Y
  Constant3 : Constant  Value=SinTable12bit_Y
  Direct Lookup Table (n-D) : LookupNDDirect  NumberOfTableDimensions=1  TableIsInput=on  Table=[4 5 6]  TableMax=[4096]
  Direct Lookup Table (n-D)1 : LookupNDDirect  NumberOfTableDimensions=1  TableIsInput=on  Table=[4 5 6]  TableMax=[4096]
  VfMDCC_EAngleCos_NULL : Outport
  VfMDCC_EAngleSin_NULL : Outport  Port=2
  wires:
  VuMDCC_MotorPositionCnt_NULL/1 -> Direct Lookup Table (n-D)/1, Direct Lookup Table (n-D)1/1
  Direct Lookup Table (n-D)/1 -> VfMDCC_EAngleCos_NULL/1
  Direct Lookup Table (n-D)1/1 -> VfMDCC_EAngleSin_NULL/1
  Constant2/1 -> Direct Lookup Table (n-D)/2
  Constant3/1 -> Direct Lookup Table (n-D)1/2

== system MDCC/DoCurCtr_sys/MDCC/UdUqCalc_Sys/MDCC_MCF_Sys/Enabled Subsystem/Harmonic_Injection_11/Subsystem/Harm_11Step_KpKi ==
  MCF_Harm_isdDes11 : Inport
  MCF_Harm_isqDes11 : Inport  Port=2
  MCF_Harm_isdAct11 : Inport  Port=3
  MCF_Harm_isqAct11 : Inport  Port=4
  Rdc_absnWoFlt_rads : Inport  Port=5
  MCF_flgHarm11PIRest : Inport  Port=6
  Harm11_KpKi_Table : Subsystem
  Harm_11Step_daxis_PI : Subsystem
  Harm_11Step_qaxis_PI : Subsystem
  MCF_Harm_ud11PI : Outport  VectorParamsAs1DForOutWhenUnconnected=off
  MCF_Harm_uq11PI : Outport  Port=2  VectorParamsAs1DForOutWhenUnconnected=off
  wires:
  MCF_Harm_isqAct11/1 -> Harm_11Step_qaxis_PI/2(MCF_Harm_isqAct11)
  MCF_Harm_isqDes11/1 -> Harm_11Step_qaxis_PI/1(MCF_Harm_isqDes11)
  MCF_Harm_isdAct11/1 -> Harm_11Step_daxis_PI/2(MCF_Harm_isdAct11)
  Harm11_KpKi_Table/2(MCF_Harm11_Ki) -> Harm_11Step_qaxis_PI/4(MCF_Harm_Ki), Harm_11Step_daxis_PI/4(MCF_Harm_Ki)
  Harm11_KpKi_Table/1(MCF_Harm11_Kp) -> Harm_11Step_qaxis_PI/3(MCF_Harm_Kp), Harm_11Step_daxis_PI/3(MCF_Harm_Kp)
  MCF_Harm_isdDes11/1 -> Harm_11Step_daxis_PI/1(MCF_Harm_isdDes11)
  Harm_11Step_qaxis_PI/1(MCF_Harm_uq11PI) -> MCF_Harm_uq11PI/1  "VfMDCC_MCF_Harm_uq11PI_V"
  Harm_11Step_daxis_PI/1(MCF_Harm_ud11PI) -> MCF_Harm_ud11PI/1  "VfMDCC_MCF_Harm_ud11PI_V"
  Rdc_absnWoFlt_rads/1 -> Harm11_KpKi_Table/1(Rdc_absnWoFlt_rads)
  MCF_flgHarm11PIRest/1 -> Harm_11Step_daxis_PI/5(MCF_flgHarm11PIRest), Harm_11Step_qaxis_PI/5(MCF_flgHarm11PIRest)

== system MDCC/DoCurCtr_sys/MDCC/UdUqCalc_Sys/MDCC_MCF_Sys/Enabled Subsystem/Harmonic_Injection_11/Subsystem/RevPark ==
  MCF_Harm_ud11PI : Inport
  MCF_Harm_uq11PI : Inport  Port=2
  MCF_Sin11Ag : Inport  Port=3
  MCF_Cos11Ag : Inport  Port=4
  Add : Sum  Inputs=+-
  Add1 : Sum
  Product{,1..3} (4 alike) : Product
  MCF_uAlpha_Harm11 : Outport  VectorParamsAs1DForOutWhenUnconnected=off
  MCF_uBeta_Harm11 : Outport  Port=2  VectorParamsAs1DForOutWhenUnconnected=off
  wires:
  Product3/1 -> Add1/2
  MCF_Harm_ud11PI/1 -> Product3/1, Product/1
  MCF_Cos11Ag/1 -> Product2/2, Product/2
  Add/1 -> MCF_uAlpha_Harm11/1
  MCF_Sin11Ag/1 -> Product1/2, Product3/2
  Add1/1 -> MCF_uBeta_Harm11/1
  MCF_Harm_uq11PI/1 -> Product2/1, Product1/1
  Product/1 -> Add/1
  Product2/1 -> Add1/1
  Product1/1 -> Add/2

== system MDCC/DoCurCtr_sys/MDCC/UdUqCalc_Sys/MDCC_MCF_Sys/Enabled Subsystem/Harmonic_Injection_13/Set_13_steps_current_isdqdes/LookUpEAngleCosSin2 ==
  VuMDCC_MotorPositionCnt_NULL : Inport  OutMin=[0]  OutMax=[4095]
  Constant2 : Constant  Value=CosTable12bit_Y
  Constant3 : Constant  Value=SinTable12bit_Y
  Direct Lookup Table (n-D) : LookupNDDirect  NumberOfTableDimensions=1  TableIsInput=on  Table=[4 5 6]  TableMax=[4096]
  Direct Lookup Table (n-D)1 : LookupNDDirect  NumberOfTableDimensions=1  TableIsInput=on  Table=[4 5 6]  TableMax=[4096]
  VfMDCC_EAngleCos_NULL : Outport
  VfMDCC_EAngleSin_NULL : Outport  Port=2
  wires:
  VuMDCC_MotorPositionCnt_NULL/1 -> Direct Lookup Table (n-D)/1, Direct Lookup Table (n-D)1/1
  Direct Lookup Table (n-D)/1 -> VfMDCC_EAngleCos_NULL/1
  Direct Lookup Table (n-D)1/1 -> VfMDCC_EAngleSin_NULL/1
  Constant2/1 -> Direct Lookup Table (n-D)/2
  Constant3/1 -> Direct Lookup Table (n-D)1/2

== system MDCC/DoCurCtr_sys/MDCC/UdUqCalc_Sys/MDCC_MCF_Sys/Enabled Subsystem/Harmonic_Injection_13/Subsystem/Harm_13Step_KpKi ==
  MCF_Harm_isdDes13 : Inport
  MCF_Harm_isqDes13 : Inport  Port=2
  MCF_Harm_isdAct13 : Inport  Port=3
  MCF_Harm_isqAct13 : Inport  Port=4
  Rdc_absnWoFlt_rads : Inport  Port=5
  MCF_flgHarm13PIRest : Inport  Port=6
  Harm13_KpKi_Table : Subsystem
  Harm_13Step_daxis_PI : Subsystem
  Harm_13Step_qaxis_PI : Subsystem
  MCF_Harm_ud13PI : Outport  VectorParamsAs1DForOutWhenUnconnected=off
  MCF_Harm_uq13PI : Outport  Port=2  VectorParamsAs1DForOutWhenUnconnected=off
  wires:
  MCF_Harm_isqAct13/1 -> Harm_13Step_qaxis_PI/2(MCF_Harm_isqAct13)
  MCF_Harm_isqDes13/1 -> Harm_13Step_qaxis_PI/1(MCF_Harm_isqDes13)
  MCF_Harm_isdAct13/1 -> Harm_13Step_daxis_PI/2(MCF_Harm_isdAct13)
  Harm13_KpKi_Table/2(MCF_Harm13_Ki) -> Harm_13Step_qaxis_PI/4(MCF_Harm_Ki), Harm_13Step_daxis_PI/4(MCF_Harm_Ki)
  Harm13_KpKi_Table/1(MCF_Harm13_Kp) -> Harm_13Step_qaxis_PI/3(MCF_Harm_Kp), Harm_13Step_daxis_PI/3(MCF_Harm_Kp)
  MCF_Harm_isdDes13/1 -> Harm_13Step_daxis_PI/1(MCF_Harm_isdDes13)
  Harm_13Step_qaxis_PI/1(MCF_Harm_uq13PI) -> MCF_Harm_uq13PI/1  "VfMDCC_MCF_Harm_uq13PI_V"
  Harm_13Step_daxis_PI/1(MCF_Harm_ud13PI) -> MCF_Harm_ud13PI/1  "VfMDCC_MCF_Harm_ud13PI_V"
  Rdc_absnWoFlt_rads/1 -> Harm13_KpKi_Table/1(Rdc_absnWoFlt_rads)
  MCF_flgHarm13PIRest/1 -> Harm_13Step_daxis_PI/5(MCF_flgHarm13PIRest), Harm_13Step_qaxis_PI/5(MCF_flgHarm13PIRest)

== system MDCC/DoCurCtr_sys/MDCC/UdUqCalc_Sys/MDCC_MCF_Sys/Enabled Subsystem/Harmonic_Injection_13/Subsystem/RevPark ==
  MCF_Harm_ud13PI : Inport
  MCF_Harm_uq13PI : Inport  Port=2
  MCF_Sin13Ag : Inport  Port=3
  MCF_Cos13Ag : Inport  Port=4
  Add : Sum  Inputs=+-
  Add1 : Sum
  Product{,1..3} (4 alike) : Product
  MCF_uAlpha_Harm13 : Outport  VectorParamsAs1DForOutWhenUnconnected=off
  MCF_uBeta_Harm13 : Outport  Port=2  VectorParamsAs1DForOutWhenUnconnected=off
  wires:
  Product3/1 -> Add1/2
  MCF_Harm_ud13PI/1 -> Product3/1, Product/1
  MCF_Cos13Ag/1 -> Product2/2, Product/2
  Add/1 -> MCF_uAlpha_Harm13/1
  MCF_Sin13Ag/1 -> Product1/2, Product3/2
  Add1/1 -> MCF_uBeta_Harm13/1
  MCF_Harm_uq13PI/1 -> Product2/1, Product1/1
  Product/1 -> Add/1
  Product2/1 -> Add1/1
  Product1/1 -> Add/2

== system MDCC/DoCurCtr_sys/MDCC/UdUqCalc_Sys/MDCC_MCF_Sys/Enabled Subsystem/Harmonic_Injection_5/Set_5_steps_current_isdqdes/LookUpEAngleCosSin2 ==
  VuMDCC_MotorPositionCnt_NULL : Inport  OutMin=[0]  OutMax=[4095]
  Constant2 : Constant  Value=CosTable12bit_Y
  Constant3 : Constant  Value=SinTable12bit_Y
  Direct Lookup Table (n-D) : LookupNDDirect  NumberOfTableDimensions=1  TableIsInput=on  Table=[4 5 6]  TableMax=[4096]
  Direct Lookup Table (n-D)1 : LookupNDDirect  NumberOfTableDimensions=1  TableIsInput=on  Table=[4 5 6]  TableMax=[4096]
  VfMDCC_EAngleCos_NULL : Outport
  VfMDCC_EAngleSin_NULL : Outport  Port=2
  wires:
  VuMDCC_MotorPositionCnt_NULL/1 -> Direct Lookup Table (n-D)/1, Direct Lookup Table (n-D)1/1
  Direct Lookup Table (n-D)/1 -> VfMDCC_EAngleCos_NULL/1
  Direct Lookup Table (n-D)1/1 -> VfMDCC_EAngleSin_NULL/1
  Constant2/1 -> Direct Lookup Table (n-D)/2
  Constant3/1 -> Direct Lookup Table (n-D)1/2

== system MDCC/DoCurCtr_sys/MDCC/UdUqCalc_Sys/MDCC_MCF_Sys/Enabled Subsystem/Harmonic_Injection_5/Subsystem/Harm_5Step_KpKi ==
  MCF_Harm_isdDes5 : Inport
  MCF_Harm_isqDes5 : Inport  Port=2
  MCF_Harm_isdAct5 : Inport  Port=3
  MCF_Harm_isqAct5 : Inport  Port=4
  Rdc_absnWoFlt_rads : Inport  Port=5
  MCF_flgHarm5PIRest : Inport  Port=6
  Harm5_KpKi_Table : Subsystem
  Harm_5Step_daxis_PI : Subsystem
  Harm_5Step_qaxis_PI : Subsystem
  MCF_Harm_ud5PI : Outport  VectorParamsAs1DForOutWhenUnconnected=off
  MCF_Harm_uq5PI : Outport  Port=2  VectorParamsAs1DForOutWhenUnconnected=off
  wires:
  MCF_Harm_isqAct5/1 -> Harm_5Step_qaxis_PI/2(MCF_Harm_isqAct5)
  MCF_Harm_isqDes5/1 -> Harm_5Step_qaxis_PI/1(MCF_Harm_isqDes5)
  MCF_Harm_isdAct5/1 -> Harm_5Step_daxis_PI/2(MCF_Harm_isdAct5)
  Harm5_KpKi_Table/2(MCF_Harm5_Ki) -> Harm_5Step_qaxis_PI/4(MCF_Harm_Ki), Harm_5Step_daxis_PI/4(MCF_Harm_Ki)
  Harm5_KpKi_Table/1(MCF_Harm5_Kp) -> Harm_5Step_qaxis_PI/3(MCF_Harm_Kp), Harm_5Step_daxis_PI/3(MCF_Harm_Kp)
  MCF_Harm_isdDes5/1 -> Harm_5Step_daxis_PI/1(MCF_Harm_isdDes5)
  Harm_5Step_qaxis_PI/1(MCF_Harm_uq5PI) -> MCF_Harm_uq5PI/1  "VfMDCC_MCF_Harm_uq5PI_V"
  Harm_5Step_daxis_PI/1(MCF_Harm_ud5PI) -> MCF_Harm_ud5PI/1  "VfMDCC_MCF_Harm_ud5PI_V"
  Rdc_absnWoFlt_rads/1 -> Harm5_KpKi_Table/1(Rdc_absnWoFlt_rads)
  MCF_flgHarm5PIRest/1 -> Harm_5Step_daxis_PI/5(MCF_flgHarm5PIRest), Harm_5Step_qaxis_PI/5(MCF_flgHarm5PIRest)

== system MDCC/DoCurCtr_sys/MDCC/UdUqCalc_Sys/MDCC_MCF_Sys/Enabled Subsystem/Harmonic_Injection_5/Subsystem/RevPark ==
  MCF_Harm_ud5PI : Inport
  MCF_Harm_uq5PI : Inport  Port=2
  MCF_Sin5Ag : Inport  Port=3
  MCF_Cos5Ag : Inport  Port=4
  Add : Sum  Inputs=+-
  Add1 : Sum
  Product{,1..3} (4 alike) : Product
  MCF_uAlpha_Harm5 : Outport  VectorParamsAs1DForOutWhenUnconnected=off
  MCF_uBeta_Harm5 : Outport  Port=2  VectorParamsAs1DForOutWhenUnconnected=off
  wires:
  Product3/1 -> Add1/2
  MCF_Harm_ud5PI/1 -> Product3/1, Product/1
  MCF_Cos5Ag/1 -> Product2/2, Product/2
  Add/1 -> MCF_uAlpha_Harm5/1
  MCF_Sin5Ag/1 -> Product1/2, Product3/2
  Add1/1 -> MCF_uBeta_Harm5/1
  MCF_Harm_uq5PI/1 -> Product2/1, Product1/1
  Product/1 -> Add/1
  Product2/1 -> Add1/1
  Product1/1 -> Add/2

== system MDCC/DoCurCtr_sys/MDCC/UdUqCalc_Sys/MDCC_MCF_Sys/Enabled Subsystem/Harmonic_Injection_7/Set_7_steps_current_isdqdes/LookUpEAngleCosSin2 ==
  VuMDCC_MotorPositionCnt_NULL : Inport  OutMin=[0]  OutMax=[4095]
  Constant2 : Constant  Value=CosTable12bit_Y
  Constant3 : Constant  Value=SinTable12bit_Y
  Direct Lookup Table (n-D) : LookupNDDirect  NumberOfTableDimensions=1  TableIsInput=on  Table=[4 5 6]  TableMax=[4096]
  Direct Lookup Table (n-D)1 : LookupNDDirect  NumberOfTableDimensions=1  TableIsInput=on  Table=[4 5 6]  TableMax=[4096]
  VfMDCC_EAngleCos_NULL : Outport
  VfMDCC_EAngleSin_NULL : Outport  Port=2
  wires:
  VuMDCC_MotorPositionCnt_NULL/1 -> Direct Lookup Table (n-D)/1, Direct Lookup Table (n-D)1/1
  Direct Lookup Table (n-D)/1 -> VfMDCC_EAngleCos_NULL/1
  Direct Lookup Table (n-D)1/1 -> VfMDCC_EAngleSin_NULL/1
  Constant2/1 -> Direct Lookup Table (n-D)/2
  Constant3/1 -> Direct Lookup Table (n-D)1/2

== system MDCC/DoCurCtr_sys/MDCC/UdUqCalc_Sys/MDCC_MCF_Sys/Enabled Subsystem/Harmonic_Injection_7/Subsystem/Harm_7Step_KpKi ==
  MCF_Harm_isdDes7 : Inport
  MCF_Harm_isqDes7 : Inport  Port=2
  MCF_Harm_isdAct7 : Inport  Port=3
  MCF_Harm_isqAct7 : Inport  Port=4
  Rdc_absnWoFlt_rads : Inport  Port=5
  MCF_flgHarm7PIRest : Inport  Port=6
  Harm7_KpKi_Table : Subsystem
  Harm_7Step_daxis_PI : Subsystem
  Harm_7Step_qaxis_PI : Subsystem
  MCF_Harm_ud7PI : Outport  VectorParamsAs1DForOutWhenUnconnected=off
  MCF_Harm_uq7PI : Outport  Port=2  VectorParamsAs1DForOutWhenUnconnected=off
  wires:
  MCF_Harm_isqAct7/1 -> Harm_7Step_qaxis_PI/2(MCF_Harm_isqAct7)
  MCF_Harm_isqDes7/1 -> Harm_7Step_qaxis_PI/1(MCF_Harm_isqDes7)
  MCF_Harm_isdAct7/1 -> Harm_7Step_daxis_PI/2(MCF_Harm_isdAct7)
  Harm7_KpKi_Table/2(MCF_Harm7_Ki) -> Harm_7Step_qaxis_PI/4(MCF_Harm_Ki), Harm_7Step_daxis_PI/4(MCF_Harm_Ki)
  Harm7_KpKi_Table/1(MCF_Harm7_Kp) -> Harm_7Step_qaxis_PI/3(MCF_Harm_Kp), Harm_7Step_daxis_PI/3(MCF_Harm_Kp)
  MCF_Harm_isdDes7/1 -> Harm_7Step_daxis_PI/1(MCF_Harm_isdDes7)
  Harm_7Step_qaxis_PI/1(MCF_Harm_uq7PI) -> MCF_Harm_uq7PI/1  "VfMDCC_MCF_Harm_uq7PI_V"
  Harm_7Step_daxis_PI/1(MCF_Harm_ud7PI) -> MCF_Harm_ud7PI/1  "VfMDCC_MCF_Harm_ud7PI_V"
  Rdc_absnWoFlt_rads/1 -> Harm7_KpKi_Table/1(Rdc_absnWoFlt_rads)
  MCF_flgHarm7PIRest/1 -> Harm_7Step_daxis_PI/5(MCF_flgHarm7PIRest), Harm_7Step_qaxis_PI/5(MCF_flgHarm7PIRest)

== system MDCC/DoCurCtr_sys/MDCC/UdUqCalc_Sys/MDCC_MCF_Sys/Enabled Subsystem/Harmonic_Injection_7/Subsystem/RevPark ==
  MCF_Harm_ud7PI : Inport
  MCF_Harm_uq7PI : Inport  Port=2
  MCF_Sin7Ag : Inport  Port=3
  MCF_Cos7Ag : Inport  Port=4
  Add : Sum  Inputs=+-
  Add1 : Sum
  Product{,1..3} (4 alike) : Product
  MCF_uAlpha_Harm7 : Outport  VectorParamsAs1DForOutWhenUnconnected=off
  MCF_uBeta_Harm7 : Outport  Port=2  VectorParamsAs1DForOutWhenUnconnected=off
  wires:
  Product3/1 -> Add1/2
  MCF_Harm_ud7PI/1 -> Product3/1, Product/1
  MCF_Cos7Ag/1 -> Product2/2, Product/2
  Add/1 -> MCF_uAlpha_Harm7/1
  MCF_Sin7Ag/1 -> Product1/2, Product3/2
  Add1/1 -> MCF_uBeta_Harm7/1
  MCF_Harm_uq7PI/1 -> Product2/1, Product1/1
  Product/1 -> Add/1
  Product2/1 -> Add1/1
  Product1/1 -> Add/2

== system MDCC/DoCurCtr_sys/MDCC/UdUqCalc_Sys/MDCC_MCF_Sys/Enabled Subsystem/Subsystem1/Park11/Subsystem ==
  In1 : Inport
  MCF_dtPWM : Inport  Port=2
  dB_Harm : Inport  Port=3
  Add : Sum
  Add1 : Sum  Inputs=-+
  Add2 : Sum
  Constant1 : Constant  OutDataTypeStr=single
  Constant2 : Constant  Value=2*pi  OutDataTypeStr=single
  Constant4 : Constant  OutDataTypeStr=single
  Divide{,1..3} (4 alike) : Product  Inputs=**
  Divide4 : Product  Inputs=*/
  Unit Delay : UnitDelay  SampleTime=-1  HasFrameUpgradeWarning=on
  Out1 : Outport
  wires:
  Add/1 -> Out1/1, Unit Delay/1
  Divide/1 -> Add/1
  Constant1/1 -> Add1/2
  Add1/1 -> Divide1/1
  Constant2/1 -> Divide2/1
  MCF_dtPWM/1 -> Divide2/2
  dB_Harm/1 -> Divide3/1
  Divide2/1 -> Divide3/2
  Divide3/1 -> Add2/2
  Constant4/1 -> Add2/1, Divide4/1
  Add2/1 -> Divide4/2
  Divide4/1 -> Divide/2, Add1/1
  In1/1 -> Divide1/2
  Divide1/1 -> Add/2
  Unit Delay/1 -> Divide/1

== system MDCC/DoCurCtr_sys/MDCC/UdUqCalc_Sys/MDCC_MCF_Sys/Enabled Subsystem/Subsystem1/Park11/Subsystem1 ==
  dB_Harm : Inport
  MCF_dtPWM : Inport  Port=2
  In1 : Inport  Port=3
  Add : Sum
  Add1 : Sum  Inputs=-+
  Add2 : Sum
  Constant1 : Constant  OutDataTypeStr=single
  Constant2 : Constant  Value=2*pi  OutDataTypeStr=single
  Constant4 : Constant  OutDataTypeStr=single
  Divide{,1..3} (4 alike) : Product  Inputs=**
  Divide4 : Product  Inputs=*/
  Unit Delay : UnitDelay  SampleTime=-1  HasFrameUpgradeWarning=on
  Out1 : Outport
  wires:
  Unit Delay/1 -> Divide/1
  Divide1/1 -> Add/2
  In1/1 -> Divide1/2
  Divide4/1 -> Add1/1, Divide/2
  Add2/1 -> Divide4/2
  Constant4/1 -> Divide4/1, Add2/1
  Divide3/1 -> Add2/2
  Divide2/1 -> Divide3/2
  dB_Harm/1 -> Divide3/1
  MCF_dtPWM/1 -> Divide2/2
  Constant2/1 -> Divide2/1
  Add1/1 -> Divide1/1
  Constant1/1 -> Add1/2
  Divide/1 -> Add/1
  Add/1 -> Unit Delay/1, Out1/1

== system MDCC/DoCurCtr_sys/MDCC/UdUqCalc_Sys/MDCC_MCF_Sys/Enabled Subsystem/Subsystem1/Park13/Subsystem ==
  In1 : Inport
  MCF_dtPWM : Inport  Port=2
  dB_Harm : Inport  Port=3
  Add : Sum
  Add1 : Sum  Inputs=-+
  Add2 : Sum
  Constant1 : Constant  OutDataTypeStr=single
  Constant2 : Constant  Value=2*pi  OutDataTypeStr=single
  Constant4 : Constant  OutDataTypeStr=single
  Divide{,1..3} (4 alike) : Product  Inputs=**
  Divide4 : Product  Inputs=*/
  Unit Delay : UnitDelay  SampleTime=-1  HasFrameUpgradeWarning=on
  Out1 : Outport
  wires:
  Add/1 -> Out1/1, Unit Delay/1
  Divide/1 -> Add/1
  Constant1/1 -> Add1/2
  Add1/1 -> Divide1/1
  Constant2/1 -> Divide2/1
  MCF_dtPWM/1 -> Divide2/2
  dB_Harm/1 -> Divide3/1
  Divide2/1 -> Divide3/2
  Divide3/1 -> Add2/2
  Constant4/1 -> Add2/1, Divide4/1
  Add2/1 -> Divide4/2
  Divide4/1 -> Divide/2, Add1/1
  In1/1 -> Divide1/2
  Divide1/1 -> Add/2
  Unit Delay/1 -> Divide/1

== system MDCC/DoCurCtr_sys/MDCC/UdUqCalc_Sys/MDCC_MCF_Sys/Enabled Subsystem/Subsystem1/Park13/Subsystem1 ==
  dB_Harm : Inport
  MCF_dtPWM : Inport  Port=2
  In1 : Inport  Port=3
  Add : Sum
  Add1 : Sum  Inputs=-+
  Add2 : Sum
  Constant1 : Constant  OutDataTypeStr=single
  Constant2 : Constant  Value=2*pi  OutDataTypeStr=single
  Constant4 : Constant  OutDataTypeStr=single
  Divide{,1..3} (4 alike) : Product  Inputs=**
  Divide4 : Product  Inputs=*/
  Unit Delay : UnitDelay  SampleTime=-1  HasFrameUpgradeWarning=on
  Out1 : Outport
  wires:
  Unit Delay/1 -> Divide/1
  Divide1/1 -> Add/2
  In1/1 -> Divide1/2
  Divide4/1 -> Add1/1, Divide/2
  Add2/1 -> Divide4/2
  Constant4/1 -> Divide4/1, Add2/1
  Divide3/1 -> Add2/2
  Divide2/1 -> Divide3/2
  dB_Harm/1 -> Divide3/1
  MCF_dtPWM/1 -> Divide2/2
  Constant2/1 -> Divide2/1
  Add1/1 -> Divide1/1
  Constant1/1 -> Add1/2
  Divide/1 -> Add/1
  Add/1 -> Unit Delay/1, Out1/1
